simulink model "pd_control_v3"  (R2022b)
settings: Solver=VariableStepAuto  StartTime=0.0  StopTime=5  RelTol=1e-3
values from neighbouring files (symbols this model uses):
  m = 6    [coordinator_v2.m]
  N = 10    [coordinator_v2.m]
undefined symbols (not defined in the file or in its folder): X, Y, Z
libraries: sm_lib x191, nesl_utility x71
(part 1 of 5)
settings Model: Creator=25394  LastModifiedBy=bijia

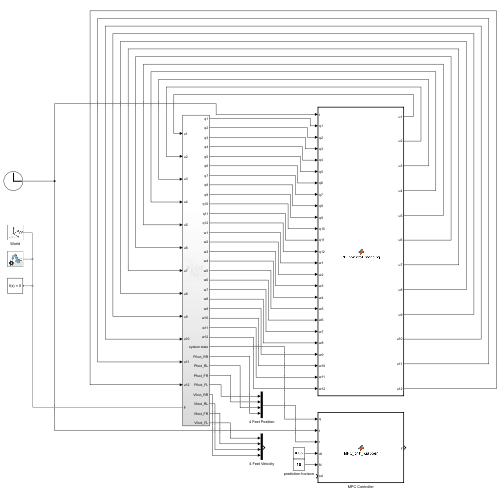
[thumbnail: Simulink's stored preview of the top-level diagram]
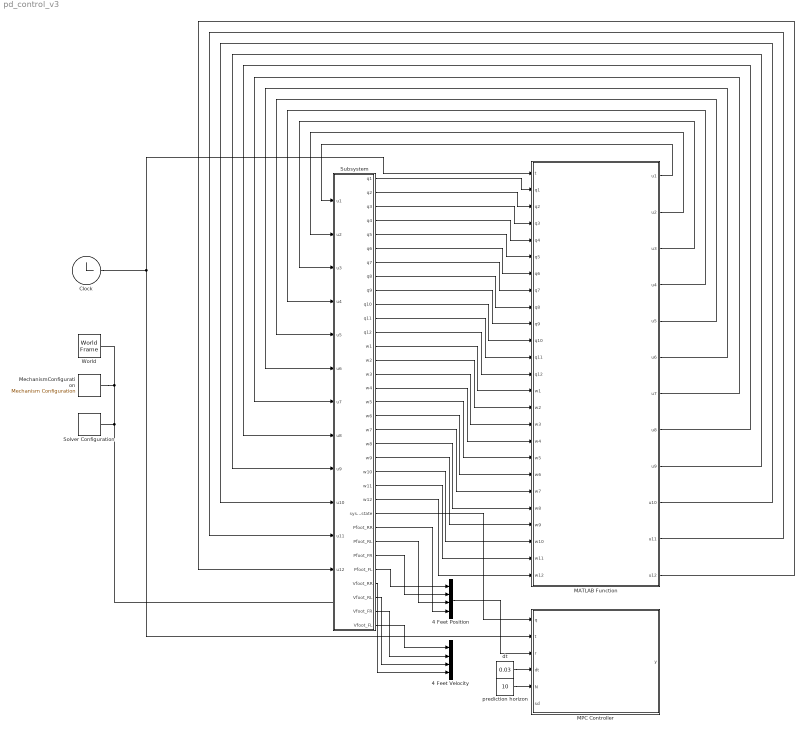
== system pd_control_v3 ==
  4 Feet Position : Mux
  4 Feet Velocity : Mux
  Clock : Clock
  MATLAB Function : MATLAB Function  TreatAsAtomicUnit=on
  MPC Controller : MATLAB Function  TreatAsAtomicUnit=on
  MechanismConfiguration : sm_lib/Utilities/Mechanism Configuration  UniformGravity=Constant  GravityVector=[0 0 -9.80665]  GravityUnits=m/s^2  LinearizationDelta=0.001  JointModeTransitionNonlinearIterations=2
  Solver Configuration : nesl_utility/Solver Configuration  PhysicalDomain=network_engine_domain  SubClassName=solver  LeftPortType=input  RightPortType=generic  Tones=[]  Harmonics=[]  SimulateNoise=off  Profile=off  UseLocalSampling=off  EnableSwitchedLinearOptims=on  FrequencyDomain=off  UseCCode=off  RelTol=0.001  AbsTol=0.001  MinStep=1e-09  ToWorkspace=off  RevertToSquareIcSolve=off  NumHomotopyIterations=100  PhasorMode=off  PhasorModeNumHarmonics=1  ConsistencySolver=NEWTON_XTOL_AFTER_FTOL  IndexReductionMethod=DerivativeReplacement  DoDC=off  ResidualTolerance=1e-09  ConsistencyTolSource=GLOBAL  ConsistencyAbsTol=0.001  ConsistencyRelTol=0.001  ConsistencyTolFactor=0.001  UseLocalSolver=off  LocalSolverChoice=NE_BACKWARD_EULER_ADVANCER  ResolveIndetEquations=on  FunctionEvalNumThread=1  LocalSolverSampleTime=0.001  DoFixedCost=off  MaxNonlinIter=3  MaxModeIter=2  ComputeImpulses=off  ImpulseIterations=2  LinearAlgebra=auto  LinearAlgebraNumThread=0  EquationFormulation=NE_TIME_EF  DelaysMemoryBudget=1024  AutomaticFiltering=on  FilteringTimeConstant=0.001  PartitionStorageMethod=AS_NEEDED  PartitionMemoryBudget=1024  PartitionMethod=ROBUST
  Subsystem : Subsystem
  World : sm_lib/Frames and Transforms/World Frame
  dt : Constant  Value=0.03
  prediction horizon : Constant  Value=10
  wires:
  Subsystem/1(q1) -> MATLAB Function/2(q1)
  Subsystem/2(q2) -> MATLAB Function/3(q2)
  Subsystem/3(q3) -> MATLAB Function/4(q3)
  Subsystem/4(q4) -> MATLAB Function/5(q4)
  Subsystem/5(q5) -> MATLAB Function/6(q5)
  Subsystem/6(q6) -> MATLAB Function/7(q6)
  Subsystem/7(q7) -> MATLAB Function/8(q7)
  Subsystem/8(q8) -> MATLAB Function/9(q8)
  Subsystem/9(q9) -> MATLAB Function/10(q9)
  Subsystem/10(q10) -> MATLAB Function/11(q10)
  Subsystem/11(q11) -> MATLAB Function/12(q11)
  Subsystem/12(q12) -> MATLAB Function/13(q12)
  Subsystem/13(w1) -> MATLAB Function/14(w1)
  Subsystem/14(w2) -> MATLAB Function/15(w2)
  Subsystem/15(w3) -> MATLAB Function/16(w3)
  Subsystem/16(w4) -> MATLAB Function/17(w4)
  Subsystem/17(w5) -> MATLAB Function/18(w5)
  Subsystem/18(w6) -> MATLAB Function/19(w6)
  Subsystem/19(w7) -> MATLAB Function/20(w7)
  Subsystem/20(w8) -> MATLAB Function/21(w8)
  Subsystem/21(w9) -> MATLAB Function/22(w9)
  Subsystem/22(w10) -> MATLAB Function/23(w10)
  Subsystem/23(w11) -> MATLAB Function/24(w11)
  Subsystem/24(w12) -> MATLAB Function/25(w12)
  MATLAB Function/1(u1) -> Subsystem/1(u1)
  MATLAB Function/2(u2) -> Subsystem/2(u2)
  MATLAB Function/3(u3) -> Subsystem/3(u3)
  MATLAB Function/4(u4) -> Subsystem/4(u4)
  MATLAB Function/5(u5) -> Subsystem/5(u5)
  MATLAB Function/6(u6) -> Subsystem/6(u6)
  MATLAB Function/7(u7) -> Subsystem/7(u7)
  MATLAB Function/8(u8) -> Subsystem/8(u8)
  MATLAB Function/9(u9) -> Subsystem/9(u9)
  MATLAB Function/12(u12) -> Subsystem/12(u12)
  MATLAB Function/10(u10) -> Subsystem/10(u10)
  MATLAB Function/11(u11) -> Subsystem/11(u11)
  Subsystem/25(system state) -> MPC Controller/1(q)
  Clock/1 -> MATLAB Function/1(t), MPC Controller/2(t)
  Subsystem/29(Pfoot_FL) -> 4 Feet Position/1
  Subsystem/28(Pfoot_FR) -> 4 Feet Position/2
  Subsystem/27(Pfoot_RL) -> 4 Feet Position/3
  Subsystem/26(Pfoot_RR) -> 4 Feet Position/4
  4 Feet Position/1 -> MPC Controller/3(r)
  dt/1 -> MPC Controller/4(dt)
  prediction horizon/1 -> MPC Controller/5(N)
  Subsystem/33(Vfoot_FL) -> 4 Feet Velocity/1
  Subsystem/32(Vfoot_FR) -> 4 Feet Velocity/2
  Subsystem/31(Vfoot_RL) -> 4 Feet Velocity/3
  Subsystem/30(Vfoot_RR) -> 4 Feet Velocity/4
  connections:
  World/RConn1 -- Subsystem/LConn1 -- Solver Configuration/RConn1 -- MechanismConfiguration/RConn1
